simulink model "ignitionScheduler"  (R2024b)
settings: Solver=VariableStepAuto  StartTime=0.0  StopTime=30  RelTol=1e-3
undefined symbols (not defined in the file or in its folder): DOWN_TABLE, DOWN_TH_BP, entity, I, initialize, p0, pressThresh, T, terminate, trigCyl, UP_TABLE, UP_TH_BP
libraries: fl_lib x32, nesl_utility x22, sdl_lib x15, simulink x1, SignalEditorBlockLib x1, engine_lib x1, autolibshared x1
(part 1 of 2)
settings Model: PauseTimes=75  Creator=Guy  LastModifiedBy=isaacito
settings SolverCC: AlgebraicLoopSolver=TrustRegion
settings DataIOCC: ReturnWorkspaceOutputs=off
settings DebuggingCC: UnconnectedInputMsg=warning  UnconnectedOutputMsg=warning  UnconnectedLineMsg=warning  PregeneratedLibrarySubsystemCodeDiagnostic=none  ArithmeticOperatorsInVariantConditions=warning
settings SFSimCC: SimUseLocalCustomCode=off  CustomCodeUndefinedFunction=UseInterfaceOnly
settings RTWCC: RTWUseLocalCustomCode=off  GPUComputeCapability=3.5
settings SimscapeCC: SimscapeNormalizeSystem=off  SimscapeLogType=all  SimscapeLogSimulationStatistics=on  SimscapeLogLimitData=off

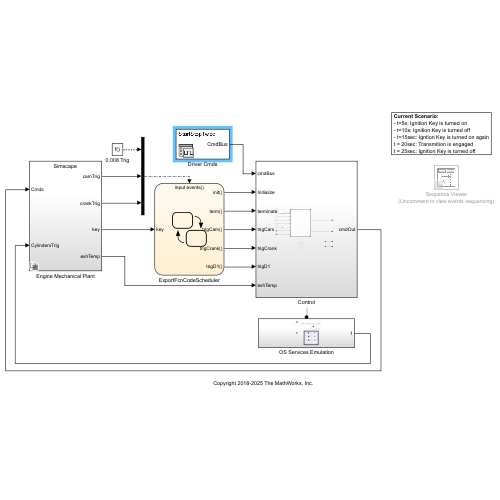
[thumbnail: Simulink's stored preview of the top-level diagram]
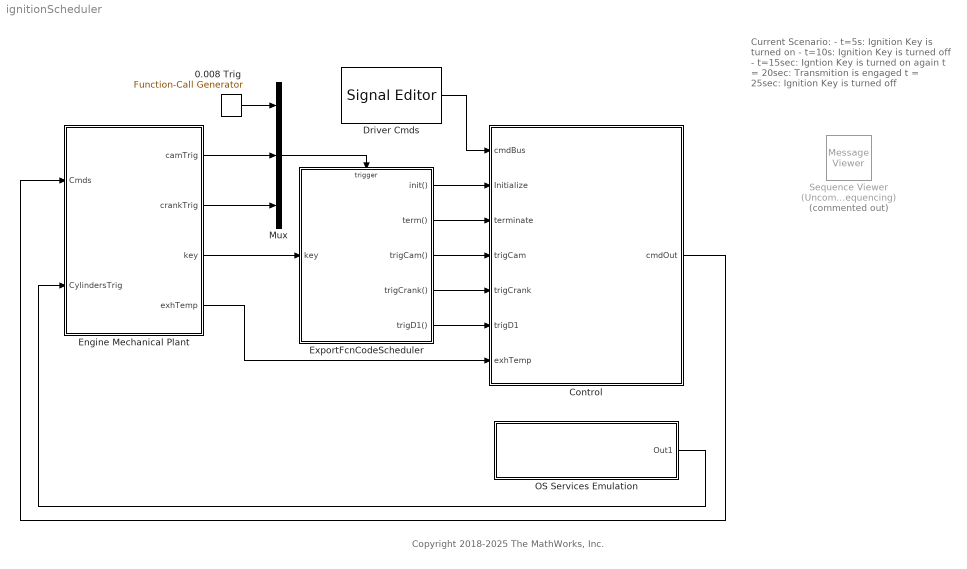
== system ignitionScheduler ==
  note: Current Scenario:
      | - t=5s: Ignition Key is turned on
      | - t=10s: Ignition Key is turned off
      | - t=15sec: Igntion Key is turned on again
      | t = 20sec: Transmition is engaged
      | t = 25sec: Ignition Key is turned off
  note: Copyright 2018-2025 The MathWorks, Inc.
  0.008 Trig : simulink/Ports & Subsystems/Function-Call Generator  sample_time=.008  numberOfIterations=1  DisallowWideOutput=off
  Control : Subsystem  VariantControl=exportFcnCode
  Driver Cmds : SignalEditorBlockLib/Signal Editor  FileName=inputScenarios.mat  ActiveScenario=StartStopTwice  ActiveSignal=CmdBus  IsBus=on  OutputBusObjectStr=Bus: opCmdBus  SampleTime=0  Interpolate=off  ZeroCross=off  OutputAfterFinalValue=Setting to zero  Unit=inherit  PreserveSignalName=on  ApplySigPropsToAllScenarios=on  ApplySigPropsToAllSignals=off
  Engine Mechanical Plant : Subsystem  Variant=on  VariantControlMode=label  LabelModeActiveChoice=SimscapeEngine
  ExportFcnCodeScheduler : Stateflow chart  TreatAsAtomicUnit=on
  Mux : Mux  Inputs=3
  OS Services Emulation : Subsystem
  Sequence Viewer (Uncomment to view events sequencing) : MessageViewer  Commented=on
  wires:
  0.008 Trig/1 -> Mux/1
  Mux/1 -> ExportFcnCodeScheduler/Trigger
  Engine Mechanical Plant/1(camTrig) -> Mux/2
  Engine Mechanical Plant/2(crankTrig) -> Mux/3
  Engine Mechanical Plant/3(key) -> ExportFcnCodeScheduler/1(key)
  Control/1(cmdOut) -> Engine Mechanical Plant/1(Cmds)
  ExportFcnCodeScheduler/1(init()) -> Control/2(Initialize)
  ExportFcnCodeScheduler/2(term()) -> Control/3(terminate)
  ExportFcnCodeScheduler/3(trigCam()) -> Control/4(trigCam)
  ExportFcnCodeScheduler/4(trigCrank()) -> Control/5(trigCrank)
  ExportFcnCodeScheduler/5(trigD1()) -> Control/6(trigD1)
  Engine Mechanical Plant/4(exhTemp) -> Control/7(exhTemp)
  OS Services Emulation/1(Out1) -> Engine Mechanical Plant/2(CylindersTrig)
  Driver Cmds/1 -> Control/1(cmdBus)

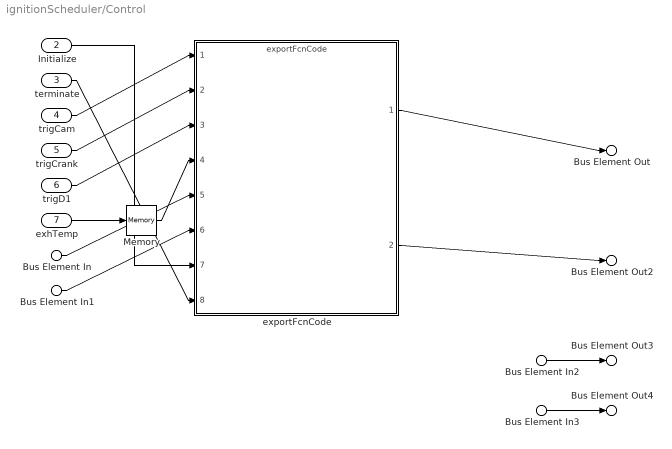
== system ignitionScheduler/Control ==
  Bus Element In1 : Inport  PortName=cmdBus  Element=Throttle
  Bus Element In3 : Inport  PortName=cmdBus  Element=EngageTransmission
  Bus Element In : Inport  PortName=cmdBus  Element=IgnitionKey
  Bus Element In2 : Inport  PortName=cmdBus  Element=IgnitionKey
  Initialize : Inport  Port=2
  terminate : Inport  Port=3
  trigCam : Inport  Port=4
  trigCrank : Inport  Port=5
  trigD1 : Inport  Port=6
  exhTemp : Inport  Port=7
  Memory : Memory
  exportFcnCode : ModelReference  ModelNameDialog=exportFcnCode.slx  SimulationMode=Normal  ShowModelInitializePort=on  ShowModelTerminatePort=on  ScheduleRates=on  ModelEventPortInfo=I:initialize,T:terminate  ModelReferenceVersion=1.150
  Bus Element Out : Outport  VectorParamsAs1DForOutWhenUnconnected=off  PortName=cmdOut  Element=starter
  Bus Element Out2 : Outport  VectorParamsAs1DForOutWhenUnconnected=off  PortName=cmdOut  Element=throttle
  Bus Element Out3 : Outport  VectorParamsAs1DForOutWhenUnconnected=off  PortName=cmdOut  Element=key
  Bus Element Out4 : Outport  VectorParamsAs1DForOutWhenUnconnected=off  PortName=cmdOut  Element=EngageTransmission
  wires:
  exportFcnCode/2 -> Bus Element Out2/1
  exportFcnCode/1 -> Bus Element Out/1
  exhTemp/1 -> Memory/1
  Bus Element In/1 -> exportFcnCode/5
  Bus Element In1/1 -> exportFcnCode/6
  Bus Element In2/1 -> Bus Element Out3/1
  Bus Element In3/1 -> Bus Element Out4/1
  Memory/1 -> exportFcnCode/4
  Initialize/1 -> exportFcnCode/7
  terminate/1 -> exportFcnCode/8
  trigCam/1 -> exportFcnCode/1
  trigCrank/1 -> exportFcnCode/2
  trigD1/1 -> exportFcnCode/3

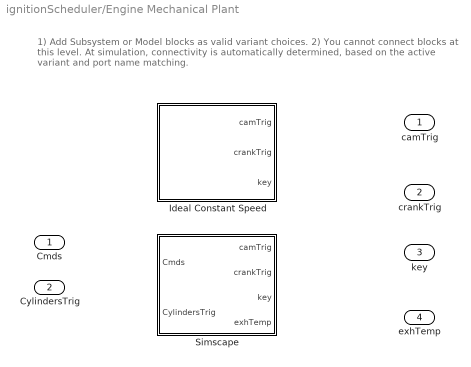
== system ignitionScheduler/Engine Mechanical Plant ==
  note: 1) Add Subsystem or Model blocks as valid variant choices.
      | 2) You cannot connect blocks at this level. At simulation, connectivity is automatically
      | determined, based on the active variant and port name matching.
  Cmds : Inport
  CylindersTrig : Inport  Port=2
  Ideal Constant Speed : Subsystem  VariantControl=idealEngine
  Simscape : Subsystem  VariantControl=SimscapeEngine
  camTrig : Outport  VectorParamsAs1DForOutWhenUnconnected=off
  crankTrig : Outport  Port=2  VectorParamsAs1DForOutWhenUnconnected=off
  key : Outport  Port=3  VectorParamsAs1DForOutWhenUnconnected=off
  exhTemp : Outport  Port=4  VectorParamsAs1DForOutWhenUnconnected=off

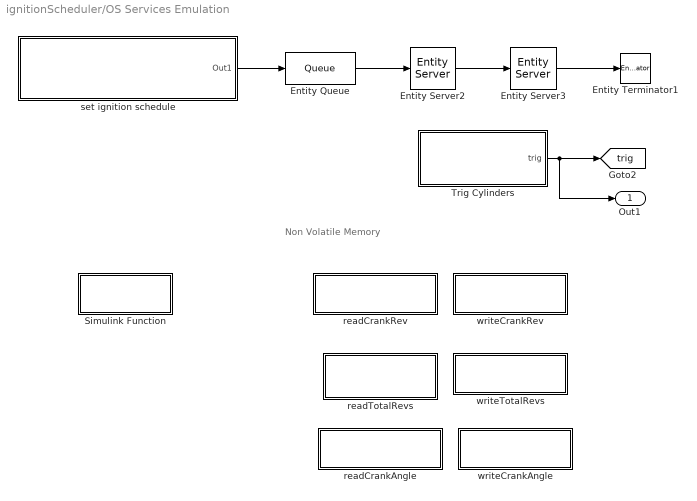
== system ignitionScheduler/OS Services Emulation ==
  note: Non Volatile Memory
  Entity Queue : Queue  InputPortMessageModes=m  OutputPortMessageModes=m  Capacity=1
  Entity Server2 : EntityServer  InputPortMessageModes=m  OutputPortMessageModes=m  Capacity=1  ServiceTimeSource=Attribute  ServiceTimeAttributeName=timeout  ServiceCompleteAction=trigCyl(entity.cyl,true);
  Entity Server3 : EntityServer  InputPortMessageModes=m  OutputPortMessageModes=m  Capacity=1  ServiceTimeSource=Attribute  ServiceTimeValue=0.01  ServiceTimeAttributeName=duration  ServiceCompleteAction=trigCyl(entity.cyl,false);
  Entity Terminator1 : EntityTerminator  InputPortMessageModes=m
  Simulink Function : Subsystem  TreatAsAtomicUnit=on
  Trig Cylinders : Subsystem  TreatAsAtomicUnit=on
  readCrankAngle : Subsystem  TreatAsAtomicUnit=on
  readCrankRev : Subsystem  TreatAsAtomicUnit=on
  readTotalRevs : Subsystem  TreatAsAtomicUnit=on
  set ignition schedule : Subsystem  TreatAsAtomicUnit=on
  writeCrankAngle : Subsystem  TreatAsAtomicUnit=on
  writeCrankRev : Subsystem  TreatAsAtomicUnit=on
  writeTotalRevs : Subsystem  TreatAsAtomicUnit=on
  Out1 : Outport  VectorParamsAs1DForOutWhenUnconnected=off
  tag scope: trig=global
  wires:
  Trig Cylinders/1(trig) -> Out1/1, [trig]
  Entity Server2/1 -> Entity Server3/1
  set ignition schedule/1(Out1) -> Entity Queue/1
  Entity Queue/1 -> Entity Server2/1
  Entity Server3/1 -> Entity Terminator1/1

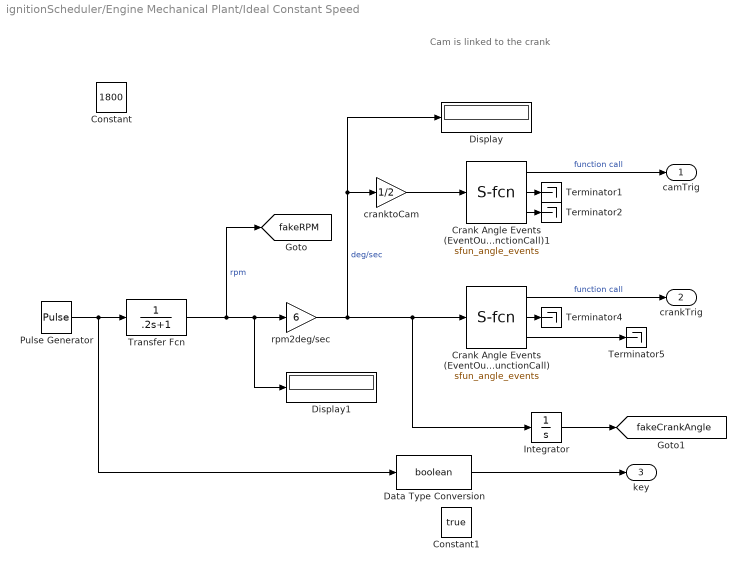
== system ignitionScheduler/Engine Mechanical Plant/Ideal Constant Speed ==
  note: Cam is linked to the crank
  Constant : Constant  Value=1800
  Constant1 : Constant  Value=true  OutDataTypeStr=boolean
  Crank Angle Events (EventOutputType: FunctionCall) : S-Function  LoadFcn=|  FunctionName=sfun_angle_events  Parameters=CrossingAngles, InitialAngle, eventOutputType, clockwiseOnly  SFunctionDeploymentMode=off  EnableBusSupport=off  mask(AnglularIntegratorWithEventDetection){CrossingAngles=[0:10:340], InitialAngle=0, EventOutputType=Function Call, ClockwiseOnly=on}
      | DVG.Registry.registerIcon(...
      | 'BlockIcon.SFunAngleEvents', ...
      | fullfile(matlabroot,'toolbox','simulink','simdemos','simfeatures','slexToothedWheel.svg'))
      mask prompts: CrossingAngles "Crossing Angles:"; InitialAngle "Initial Angle:"; EventOutputType "Event output type:"; ClockwiseOnly "Assume clockwise rotation only"
      mask help:
      | This block integrates the angular velocity input to compute the angle and to fire events at the specified crossing angles. All angles are in degrees, with 0 at the top, incresing clockwise.
      |
      | The crossings angles should be specified as a monotonically increasing vector, with the first element set to 0 and the last element being less than 360 degrees.
      |
      | The first output is a function call, which is fired when an angle crossing event is detected.
      |
      | The second output indicates the direction of the angle crossing event, true for clockwise and false for anti-clockwise.
      |
      | The third output is the angle, wrapped to be in [0, 360) degrees.
      mask init:
      | clockwiseOnly = isequal(get_param(gcb,'ClockwiseOnly'),'on');
      | 
      | switch get_param(gcb,'EventOutputType')
      |     case 'Trigger Pulse'
      |         eventOutputType = 0;
      |     case 'Function Call'
      |         eventOutputType = 1;
      |     otherwise
      |         eventOutputType = 2;
      | end
      mask TypeOptions EventOutputType: Trigger Pulse | Function Call
      mask Display: %image('slexToothedWheel.svg');
  Crank Angle Events (EventOutputType: FunctionCall)1 : S-Function  LoadFcn=|  FunctionName=sfun_angle_events  Parameters=CrossingAngles, InitialAngle, eventOutputType, clockwiseOnly  SFunctionDeploymentMode=off  EnableBusSupport=off  mask(AnglularIntegratorWithEventDetection){CrossingAngles=[0 ], InitialAngle=320, EventOutputType=Function Call, ClockwiseOnly=on}
      | DVG.Registry.registerIcon(...
      | 'BlockIcon.SFunAngleEvents', ...
      | fullfile(matlabroot,'toolbox','simulink','simdemos','simfeatures','slexToothedWheel.svg'))
      mask prompts: CrossingAngles "Crossing Angles:"; InitialAngle "Initial Angle:"; EventOutputType "Event output type:"; ClockwiseOnly "Assume clockwise rotation only"
      mask help:
      | This block integrates the angular velocity input to compute the angle and to fire events at the specified crossing angles. All angles are in degrees, with 0 at the top, incresing clockwise.
      |
      | The crossings angles should be specified as a monotonically increasing vector, with the first element set to 0 and the last element being less than 360 degrees.
      |
      | The first output is a function call, which is fired when an angle crossing event is detected.
      |
      | The second output indicates the direction of the angle crossing event, true for clockwise and false for anti-clockwise.
      |
      | The third output is the angle, wrapped to be in [0, 360) degrees.
      mask init: same as ignitionScheduler/Engine Mechanical Plant/Ideal Constant Speed/Crank Angle Events (EventOutputType: FunctionCall)
      mask TypeOptions EventOutputType: Trigger Pulse | Function Call
      mask Display: %image('slexToothedWheel.svg');
  Data Type Conversion : DataTypeConversion  OutDataTypeStr=boolean  SaturateOnIntegerOverflow=off  RndMeth=Floor
  Display : Display
  Display1 : Display
  Integrator : Integrator  WrapState=on  WrappedStateUpperValue=720  WrappedStateLowerValue=0
  Pulse Generator : DiscretePulseGenerator  PulseType=Time based  Amplitude=1000  Period=100 %6.123  PulseWidth=50  PhaseDelay=1
  Terminator{1..2,4..5} (4 alike) : Terminator
  Transfer Fcn : TransferFcn  Denominator=[.2 1]
  cranktoCam : Gain  Gain=1/2
  rpm2deg/sec : Gain  Gain=6
  camTrig : Outport  VectorParamsAs1DForOutWhenUnconnected=off
  crankTrig : Outport  Port=2  VectorParamsAs1DForOutWhenUnconnected=off
  key : Outport  Port=3  VectorParamsAs1DForOutWhenUnconnected=off
  tag scope: fakeCrankAngle=global, fakeRPM=global
  wires:
  Crank Angle Events (EventOutputType: FunctionCall)1/3 -> Terminator2/1
  Crank Angle Events (EventOutputType: FunctionCall)/3 -> Terminator5/1
  Transfer Fcn/1 -> [fakeRPM], Display1/1, rpm2deg/sec/1  "rpm"
  rpm2deg/sec/1 -> Integrator/1, Crank Angle Events (EventOutputType: FunctionCall)/1, cranktoCam/1, Display/1  "deg/sec"
  Crank Angle Events (EventOutputType: FunctionCall)/2 -> Terminator4/1
  Crank Angle Events (EventOutputType: FunctionCall)/1 -> crankTrig/1  "function call"
  Crank Angle Events (EventOutputType: FunctionCall)1/2 -> Terminator1/1
  cranktoCam/1 -> Crank Angle Events (EventOutputType: FunctionCall)1/1
  Crank Angle Events (EventOutputType: FunctionCall)1/1 -> camTrig/1  "function call"
  Data Type Conversion/1 -> key/1
  Pulse Generator/1 -> Data Type Conversion/1, Transfer Fcn/1
  Integrator/1 -> [fakeCrankAngle]

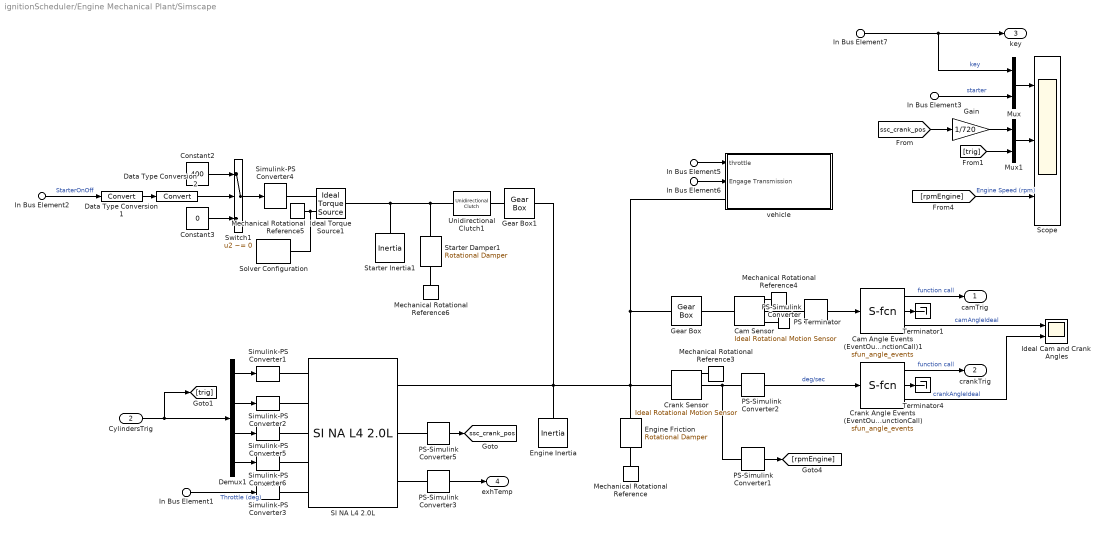
== system ignitionScheduler/Engine Mechanical Plant/Simscape ==
  In Bus Element1 : Inport  PortName=Cmds  Element=throttle
  In Bus Element5 : Inport  PortName=Cmds  Element=throttle
  In Bus Element6 : Inport  PortName=Cmds  Element=EngageTransmission
  In Bus Element7 : Inport  PortName=Cmds  Element=key
  In Bus Element2 : Inport  PortName=Cmds  Element=starter
  In Bus Element3 : Inport  PortName=Cmds  Element=starter
  CylindersTrig : Inport  Port=2
  Cam Angle Events (EventOutputType: FunctionCall)1 : S-Function  LoadFcn=|  FunctionName=sfun_angle_events  Parameters=CrossingAngles, InitialAngle, eventOutputType, clockwiseOnly  SFunctionDeploymentMode=off  EnableBusSupport=off  mask(AnglularIntegratorWithEventDetection){CrossingAngles=[0 ], InitialAngle=320, EventOutputType=Function Call, ClockwiseOnly=on}
      | DVG.Registry.registerIcon(...
      | 'BlockIcon.SFunAngleEvents', ...
      | fullfile(matlabroot,'toolbox','simulink','simdemos','simfeatures','slexToothedWheel.svg'))
      mask prompts: CrossingAngles "Crossing Angles:"; InitialAngle "Initial Angle:"; EventOutputType "Event output type:"; ClockwiseOnly "Assume clockwise rotation only"
      mask help:
      | This block integrates the angular velocity input to compute the angle and to fire events at the specified crossing angles. All angles are in degrees, with 0 at the top, incresing clockwise.
      |
      | The crossings angles should be specified as a monotonically increasing vector, with the first element set to 0 and the last element being less than 360 degrees.
      |
      | The first output is a function call, which is fired when an angle crossing event is detected.
      |
      | The second output indicates the direction of the angle crossing event, true for clockwise and false for anti-clockwise.
      |
      | The third output is the angle, wrapped to be in [0, 360) degrees.
      mask init: same as ignitionScheduler/Engine Mechanical Plant/Ideal Constant Speed/Crank Angle Events (EventOutputType: FunctionCall)
      mask TypeOptions EventOutputType: Trigger Pulse | Function Call
      mask Display: %image('slexToothedWheel.svg');
  Cam Sensor : fl_lib/Mechanical/Mechanical Sensors/Ideal Rotational Motion Sensor  reference=foundation.enum.MeasurementReference.difference  acceleration_port=false  velocity_port=true  position_port=true  wrap_angle=simscape.enum.onoff.off  offset=0 rad
  Constant2 : Constant  Value=400
  Constant3 : Constant  Value=0
  Crank Angle Events (EventOutputType: FunctionCall) : S-Function  LoadFcn=|  FunctionName=sfun_angle_events  Parameters=CrossingAngles, InitialAngle, eventOutputType, clockwiseOnly  SFunctionDeploymentMode=off  EnableBusSupport=off  mask(AnglularIntegratorWithEventDetection){CrossingAngles=[0:10:340], InitialAngle=0, EventOutputType=Function Call, ClockwiseOnly=on}
      | DVG.Registry.registerIcon(...
      | 'BlockIcon.SFunAngleEvents', ...
      | fullfile(matlabroot,'toolbox','simulink','simdemos','simfeatures','slexToothedWheel.svg'))
      mask prompts: CrossingAngles "Crossing Angles:"; InitialAngle "Initial Angle:"; EventOutputType "Event output type:"; ClockwiseOnly "Assume clockwise rotation only"
      mask help:
      | This block integrates the angular velocity input to compute the angle and to fire events at the specified crossing angles. All angles are in degrees, with 0 at the top, incresing clockwise.
      |
      | The crossings angles should be specified as a monotonically increasing vector, with the first element set to 0 and the last element being less than 360 degrees.
      |
      | The first output is a function call, which is fired when an angle crossing event is detected.
      |
      | The second output indicates the direction of the angle crossing event, true for clockwise and false for anti-clockwise.
      |
      | The third output is the angle, wrapped to be in [0, 360) degrees.
      mask init: same as ignitionScheduler/Engine Mechanical Plant/Ideal Constant Speed/Crank Angle Events (EventOutputType: FunctionCall)
      mask TypeOptions EventOutputType: Trigger Pulse | Function Call
      mask Display: %image('slexToothedWheel.svg');
  Crank Sensor : fl_lib/Mechanical/Mechanical Sensors/Ideal Rotational Motion Sensor  reference=foundation.enum.MeasurementReference.difference  acceleration_port=false  velocity_port=true  position_port=true  wrap_angle=simscape.enum.onoff.off  offset=0 rad
  Data Type Conversion1 : DataTypeConversion  SaturateOnIntegerOverflow=off  RndMeth=Floor
  Data Type Conversion2 : DataTypeConversion  SaturateOnIntegerOverflow=off  RndMeth=Floor
  Demux1 : Demux
  Engine Friction : fl_lib/Mechanical/Rotational Elements/Rotational Damper  D=0.06 m*N/rpm  w_specify=off  w_priority=None  w=0 rad/s  w_nominal_specify=off  w_nominal_value=1  w_nominal_unit=rad/s  t_specify=off  t_priority=None  t=0 N*m  t_nominal_specify=off  t_nominal_value=1  t_nominal_unit=N*m
      settings: AttributesFormatString=|
      | %<D>
      | %<D_unit>
  Engine Inertia : fl_lib/Mechanical/Rotational Elements/Inertia  inertia=0.24 kg*m^2  num_ports=foundation.enum.numPorts2.one  w_specify=off  w_priority=High  w=0 rad/s  w_nominal_specify=off  w_nominal_value=1  w_nominal_unit=rad/s  t_specify=off  t_priority=None  t=0 N*m  t_nominal_specify=off  t_nominal_value=1  t_nominal_unit=N*m
      settings: AttributesFormatString=|
      | %<inertia>
      | %<inertia_unit>
      | %<w_specify>
  Gain : Gain  Gain=1/720
  Gear Box : fl_lib/Mechanical/Mechanisms/Gear Box  ratio=2  t_in_specify=off  t_in_priority=None  t_in=0 N*m  t_in_nominal_specify=off  t_in_nominal_value=1  t_in_nominal_unit=N*m  t_out_specify=off  t_out_priority=None  t_out=0 N*m  t_out_nominal_specify=off  t_out_nominal_value=1  t_out_nominal_unit=N*m
  Gear Box1 : fl_lib/Mechanical/Mechanisms/Gear Box  ratio=20  t_in_specify=off  t_in_priority=None  t_in=0 N*m  t_in_nominal_specify=off  t_in_nominal_value=1  t_in_nominal_unit=N*m  t_out_specify=off  t_out_priority=None  t_out=0 N*m  t_out_nominal_specify=off  t_out_nominal_value=1  t_out_nominal_unit=N*m
      settings: AttributesFormatString=%<ratio>
  Ideal Cam and Crank Angles : Scope  NumInputPorts=2
  Ideal Torque Source1 : fl_lib/Mechanical/Mechanical Sources/Ideal Torque Source
  Mechanical Rotational Reference{,3..6} (5 alike) : fl_lib/Mechanical/Rotational Elements/Mechanical Rotational Reference
  Mux : Mux  Inputs=2
  Mux1 : Mux  Inputs=2
  PS Terminator : fl_lib/Physical Signals/Sinks/PS Terminator
  PS-Simulink Converter : nesl_utility/PS-Simulink Converter  PhysicalDomain=network_engine_domain  SubClassName=ps_output  LeftPortType=input  RightPortType=output  PseudoPeriodic=off  Frequencies=[]  VectorFormat=1-D array  Unit=deg/s  AffineConversion=off
  PS-Simulink Converter1 : nesl_utility/PS-Simulink Converter  PhysicalDomain=network_engine_domain  SubClassName=ps_output  LeftPortType=input  RightPortType=output  PseudoPeriodic=off  Frequencies=[]  VectorFormat=1-D array  Unit=rpm  AffineConversion=off
  PS-Simulink Converter2 : nesl_utility/PS-Simulink Converter  PhysicalDomain=network_engine_domain  SubClassName=ps_output  LeftPortType=input  RightPortType=output  PseudoPeriodic=off  Frequencies=[]  VectorFormat=1-D array  Unit=deg/s  AffineConversion=off
  PS-Simulink Converter3 : nesl_utility/PS-Simulink Converter  PhysicalDomain=network_engine_domain  SubClassName=ps_output  LeftPortType=input  RightPortType=output  PseudoPeriodic=off  Frequencies=[]  VectorFormat=1-D array  Unit=degC  AffineConversion=on
  PS-Simulink Converter5 : nesl_utility/PS-Simulink Converter  PhysicalDomain=network_engine_domain  SubClassName=ps_output  LeftPortType=input  RightPortType=output  PseudoPeriodic=off  Frequencies=[]  VectorFormat=1-D array  Unit=deg  AffineConversion=off
  SI NA L4 2.0L : engine_lib/SI NA L4 2.0L
      settings: InternalSimscapePortConfiguration="{\"Bottom\":[],\"Left\":[{\"id\":\"ig1\",\"label\":\"ig1\",\"type\":\"input\"},{\"id\":\"ig2\",\"label\":\"ig2\",\"type\":\"input\"},{\"id\":\"ig3\",\"label\":\"ig3\",\"type\":\"input\"},{\"id\":\"ig4\",\"label\":\"ig4\",\"type\":\"input\"},{\"id\":\"thr_cmd\",\"label\":\"THR\",\"type\":\"input\"}],\"Right\":[{\"id\":\"R\",\"label\":\"R\",\"type\":\"foundation.mechanical.rotational.rotational\"},{\"id\":\"crkpos\",\"label\":\"cpos\",\"type\":\"output\"},{\"id\":\"T_exwall\",\"label\":\"Tew\",\"type\":\"output\"}],\"Top\":[]}"
  Scope : Scope  NumInputPorts=3
  Simulink-PS Converter{1..2,5..6} (4 alike) : nesl_utility/Simulink-PS Converter  PhysicalDomain=network_engine_domain  SubClassName=ps_input  LeftPortType=input  RightPortType=output  PseudoPeriodic=off  Frequencies=[]  NoiseDistribution=none  NoiseParameters=[]  Unit=1  AffineConversion=off  FilteringAndDerivatives=provide  SimscapeFilterOrder=1  InputFilterTimeConstant=0.001  UdotUserProvided=0
  Simulink-PS Converter3 : nesl_utility/Simulink-PS Converter  PhysicalDomain=network_engine_domain  SubClassName=ps_input  LeftPortType=input  RightPortType=output  PseudoPeriodic=off  Frequencies=[]  NoiseDistribution=none  NoiseParameters=[]  Unit=deg  AffineConversion=off  FilteringAndDerivatives=provide  SimscapeFilterOrder=1  InputFilterTimeConstant=0.001  UdotUserProvided=0
  Simulink-PS Converter4 : nesl_utility/Simulink-PS Converter  PhysicalDomain=network_engine_domain  SubClassName=ps_input  LeftPortType=input  RightPortType=output  PseudoPeriodic=off  Frequencies=[]  NoiseDistribution=none  NoiseParameters=[]  Unit=N*m  AffineConversion=off  FilteringAndDerivatives=filter  SimscapeFilterOrder=1  InputFilterTimeConstant=0.001  UdotUserProvided=1
  Solver Configuration : nesl_utility/Solver Configuration  PhysicalDomain=network_engine_domain  SubClassName=solver  LeftPortType=input  RightPortType=generic  Tones=[]  Harmonics=[]  SimulateNoise=off  Profile=off  UseLocalSampling=off  EnableSwitchedLinearOptims=on  FrequencyDomain=off  UseCCode=off  RelTol=0.001  AbsTol=1e-06  MinStep=1e-09  ToWorkspace=off  RevertToSquareIcSolve=off  NumHomotopyIterations=100  PhasorMode=off  PhasorModeNumHarmonics=1  ConsistencySolver=NEWTON_FTOL  IndexReductionMethod=DerivativeReplacement  DoDC=off  ResidualTolerance=1e-09  ConsistencyTolSource=GLOBAL  ConsistencyAbsTol=0.001  ConsistencyRelTol=0.001  ConsistencyTolFactor=0.001  UseLocalSolver=off  LocalSolverChoice=NE_BACKWARD_EULER_ADVANCER  ResolveIndetEquations=on  FunctionEvalNumThread=1  LocalSolverSampleTime=0.001  DoFixedCost=off  MaxNonlinIter=3  MaxModeIter=2  ComputeImpulses=off  ImpulseIterations=2  LinearAlgebra=Sparse  LinearAlgebraNumThread=0  EquationFormulation=NE_TIME_EF  DelaysMemoryBudget=1024  AutomaticFiltering=on  FilteringTimeConstant=0.001  PartitionStorageMethod=AS_NEEDED  PartitionMemoryBudget=1024  PartitionMethod=FAST  MultibodyUseLocalSolver=off  MultibodyLocalSolverChoice=ODE1  MultibodyLocalSolverSampleTime=0.001
      settings: AttributesFormatString=Local solver %<UseLocalSolver>
  Starter Damper1 : fl_lib/Mechanical/Rotational Elements/Rotational Damper  D=0.1 m*N/rpm  w_specify=off  w_priority=None  w=0 rad/s  w_nominal_specify=off  w_nominal_value=1  w_nominal_unit=rad/s  t_specify=off  t_priority=None  t=0 N*m  t_nominal_specify=off  t_nominal_value=1  t_nominal_unit=N*m
      settings: AttributesFormatString=|
      | %<D>
      | %<D_unit>
  Starter Inertia1 : fl_lib/Mechanical/Rotational Elements/Inertia  inertia=30 m^2*g  num_ports=foundation.enum.numPorts2.one  w_specify=off  w_priority=High  w=0 rad/s  w_nominal_specify=off  w_nominal_value=1  w_nominal_unit=rad/s  t_specify=off  t_priority=None  t=0 N*m  t_nominal_specify=off  t_nominal_value=1  t_nominal_unit=N*m
      settings: AttributesFormatString=|
      | %<inertia>
      | %<inertia_unit>
  Switch1 : Switch  Criteria=u2 ~= 0  SaturateOnIntegerOverflow=off  InputSameDT=off
  Terminator1 : Terminator
  Terminator4 : Terminator
  Unidirectional Clutch1 : sdl_lib/Clutches/Unidirectional Clutch  transmission_direction=1  initial_state_locked=0
      settings: InternalSimscapePortConfiguration="{\"Bottom\":[],\"Left\":[{\"id\":\"H\",\"label\":\"H\",\"type\":\"foundation.mechanical.rotational.rotational\"}],\"Right\":[{\"id\":\"R\",\"label\":\"R\",\"type\":\"foundation.mechanical.rotational.rotational\"}],\"Top\":[]}"
  vehicle : Subsystem
  camTrig : Outport  VectorParamsAs1DForOutWhenUnconnected=off
  crankTrig : Outport  Port=2  VectorParamsAs1DForOutWhenUnconnected=off
  key : Outport  Port=3  VectorParamsAs1DForOutWhenUnconnected=off
  exhTemp : Outport  Port=4  VectorParamsAs1DForOutWhenUnconnected=off
  tag scope: ssc_crank_pos=global
  wires:
  Cam Angle Events (EventOutputType: FunctionCall)1/3 -> Ideal Cam and Crank Angles/1  "camAngleIdeal"
  Crank Angle Events (EventOutputType: FunctionCall)/1 -> crankTrig/1  "function call"
  Cam Angle Events (EventOutputType: FunctionCall)1/1 -> camTrig/1  "function call"
  Crank Angle Events (EventOutputType: FunctionCall)/3 -> Ideal Cam and Crank Angles/2  "crankAngleIdeal"
  Cam Angle Events (EventOutputType: FunctionCall)1/2 -> Terminator1/1
  Crank Angle Events (EventOutputType: FunctionCall)/2 -> Terminator4/1
  PS-Simulink Converter/1 -> Cam Angle Events (EventOutputType: FunctionCall)1/1
  PS-Simulink Converter1/1 -> [rpmEngine]
  Mux/1 -> Scope/1
  [rpmEngine] -> Scope/3  "Engine Speed (rpm)"
  PS-Simulink Converter2/1 -> Crank Angle Events (EventOutputType: FunctionCall)/1  "deg/sec"
  CylindersTrig/1 -> [trig], Demux1/1
  Gain/1 -> Mux1/1
  [ssc_crank_pos] -> Gain/1
  [trig] -> Mux1/2
  Mux1/1 -> Scope/2
  In Bus Element3/1 -> Mux/2  "starter"
  In Bus Element5/1 -> vehicle/1(throttle)
  In Bus Element6/1 -> vehicle/2(Engage Transmission)
  In Bus Element7/1 -> Mux/1, key/1  "key"
  In Bus Element1/1 -> Simulink-PS Converter3/1  "Throttle (deg)"
  In Bus Element2/1 -> Data Type Conversion1/1  "StarterOnOff"
  PS-Simulink Converter5/1 -> [ssc_crank_pos]
  PS-Simulink Converter3/1 -> exhTemp/1
  Data Type Conversion1/1 -> Data Type Conversion2/1
  Switch1/1 -> Simulink-PS Converter4/1
  Data Type Conversion2/1 -> Switch1/2
  Constant2/1 -> Switch1/1
  Demux1/3 -> Simulink-PS Converter5/1
  Demux1/1 -> Simulink-PS Converter1/1
  Constant3/1 -> Switch1/3
  Demux1/2 -> Simulink-PS Converter2/1
  Demux1/4 -> Simulink-PS Converter6/1
  connections:
  Mechanical Rotational Reference/LConn1 -- Engine Friction/RConn1
  Gear Box/RConn1 -- Cam Sensor/LConn1
  Mechanical Rotational Reference4/LConn1 -- Cam Sensor/RConn1
  PS-Simulink Converter/LConn1 -- Cam Sensor/RConn2
  PS Terminator/LConn1 -- Cam Sensor/RConn3
  PS-Simulink Converter2/LConn1 -- PS-Simulink Converter1/LConn1 -- Crank Sensor/RConn2
  Mechanical Rotational Reference3/LConn1 -- Crank Sensor/RConn1
  Gear Box1/RConn1 -- SI NA L4 2.0L/RConn1 -- Crank Sensor/LConn1 -- Engine Friction/LConn1 -- vehicle/LConn1 -- Gear Box/LConn1 -- Engine Inertia/LConn1
  Unidirectional Clutch1/LConn1 -- Starter Damper1/LConn1 -- Ideal Torque Source1/LConn1 -- Starter Inertia1/LConn1
  SI NA L4 2.0L/LConn5 -- Simulink-PS Converter3/RConn1
  Mechanical Rotational Reference6/LConn1 -- Starter Damper1/RConn1
  Gear Box1/LConn1 -- Unidirectional Clutch1/RConn1
  Mechanical Rotational Reference5/LConn1 -- Solver Configuration/RConn1 -- Ideal Torque Source1/RConn2
  SI NA L4 2.0L/LConn4 -- Simulink-PS Converter6/RConn1
  SI NA L4 2.0L/RConn2 -- PS-Simulink Converter5/LConn1
  SI NA L4 2.0L/LConn2 -- Simulink-PS Converter2/RConn1
  SI NA L4 2.0L/RConn3 -- PS-Simulink Converter3/LConn1
  SI NA L4 2.0L/LConn1 -- Simulink-PS Converter1/RConn1
  SI NA L4 2.0L/LConn3 -- Simulink-PS Converter5/RConn1
  Ideal Torque Source1/RConn1 -- Simulink-PS Converter4/RConn1

== system ignitionScheduler/OS Services Emulation/Simulink Function ==
  getTime : TriggerPort  TriggerType=function-call  IsSimulinkFunction=on  FunctionName=getTime  VariantControl=(inherit)
  Digital Clock : DigitalClock  SampleTime=-1
  y : ArgOut  DisableCoverage=on  ArgumentName=y
  wires:
  Digital Clock/1 -> y/1

== system ignitionScheduler/OS Services Emulation/Trig Cylinders ==
  trigCyl : TriggerPort  TriggerType=function-call  IsSimulinkFunction=on  FunctionName=trigCyl  FunctionVisibility=scoped  VariantControl=(inherit)
  Assignment : Assignment  DiagnosticForDimensions=Warning  IndexOptions=Index vector (port)  Indices=1  OutputSizes=1
  Constant : Constant  Value=[0 0 0 0]
  cyl : ArgIn  ArgumentName=cyl
  enable : ArgIn  Port=2  ArgumentName=enable
  trig : Outport  VectorParamsAs1DForOutWhenUnconnected=off
  wires:
  Constant/1 -> Assignment/1
  Assignment/1 -> trig/1
  enable/1 -> Assignment/2
  cyl/1 -> Assignment/3

== system ignitionScheduler/OS Services Emulation/readCrankAngle ==
  readCrankAngle : TriggerPort  TriggerType=function-call  IsSimulinkFunction=on  FunctionName=readCrankAngle  VariantControl=(inherit)
  Data Store Read : DataStoreRead  DataStoreName=crankAngle  IndexOptions=Index vector (dialog)  Indices=1  OutputSizes=1
  y : ArgOut  DisableCoverage=on  ArgumentName=y
  wires:
  Data Store Read/1 -> y/1

== system ignitionScheduler/OS Services Emulation/readCrankRev ==
  readCrankRev : TriggerPort  TriggerType=function-call  IsSimulinkFunction=on  FunctionName=readCrankRev  VariantControl=(inherit)
  Data Store Read : DataStoreRead  DataStoreName=rev  IndexOptions=Index vector (dialog)  Indices=1  OutputSizes=1
  y : ArgOut  DisableCoverage=on  OutDataTypeStr=boolean  ArgumentName=y
  wires:
  Data Store Read/1 -> y/1

== system ignitionScheduler/OS Services Emulation/readTotalRevs ==
  readTotalRevs : TriggerPort  TriggerType=function-call  IsSimulinkFunction=on  FunctionName=readTotalRevs  VariantControl=(inherit)
  Data Store Read : DataStoreRead  DataStoreName=totalRevs  IndexOptions=Index vector (dialog)  Indices=1  OutputSizes=1
  y : ArgOut  DisableCoverage=on  ArgumentName=y
  wires:
  Data Store Read/1 -> y/1

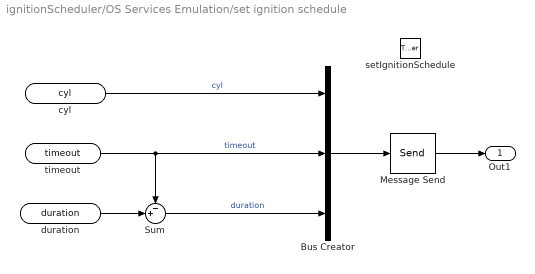
== system ignitionScheduler/OS Services Emulation/set ignition schedule ==
  setIgnitionSchedule : TriggerPort  TriggerType=function-call  IsSimulinkFunction=on  FunctionName=setIgnitionSchedule  VariantControl=(inherit)
  Bus Creator : BusCreator  Inputs=3  OutDataTypeStr=Bus: timerBus  NonVirtualBus=on
  Message Send : Send  OutputPortMessageModes=m
  Sum : Sum  Inputs=-+|
  cyl : ArgIn  ArgumentName=cyl
  timeout : ArgIn  DisableCoverage=on  Port=2  ArgumentName=timeout
  duration : ArgIn  Port=3  ArgumentName=duration
  Out1 : Outport  VectorParamsAs1DForOutWhenUnconnected=off
  wires:
  Message Send/1 -> Out1/1
  cyl/1 -> Bus Creator/1  "cyl"
  Sum/1 -> Bus Creator/3  "duration"
  duration/1 -> Sum/2
  timeout/1 -> Sum/1, Bus Creator/2  "timeout"
  Bus Creator/1 -> Message Send/1

== system ignitionScheduler/OS Services Emulation/writeCrankAngle ==
  writeCrankAngle : TriggerPort  TriggerType=function-call  IsSimulinkFunction=on  FunctionName=writeCrankAngle  VariantControl=(inherit)
  Data Store Write : DataStoreWrite  DataStoreName=crankAngle  IndexOptions=Index vector (dialog)  Indices=1  OutputSizes=1
  u : ArgIn  DisableCoverage=on  ArgumentName=u
  wires:
  u/1 -> Data Store Write/1

== system ignitionScheduler/OS Services Emulation/writeCrankRev ==
  writeCrankRev : TriggerPort  TriggerType=function-call  IsSimulinkFunction=on  FunctionName=writeCrankRev  VariantControl=(inherit)
  Data Store Write : DataStoreWrite  DataStoreName=rev  IndexOptions=Index vector (dialog)  Indices=1  OutputSizes=1
  u : ArgIn  DisableCoverage=on  OutDataTypeStr=boolean  ArgumentName=u
  wires:
  u/1 -> Data Store Write/1

== system ignitionScheduler/OS Services Emulation/writeTotalRevs ==
  writeTotalRevs : TriggerPort  TriggerType=function-call  IsSimulinkFunction=on  FunctionName=writeTotalRevs  VariantControl=(inherit)
  Data Store Write : DataStoreWrite  DataStoreName=totalRevs  IndexOptions=Index vector (dialog)  Indices=1  OutputSizes=1
  u : ArgIn  DisableCoverage=on  ArgumentName=u
  wires:
  u/1 -> Data Store Write/1

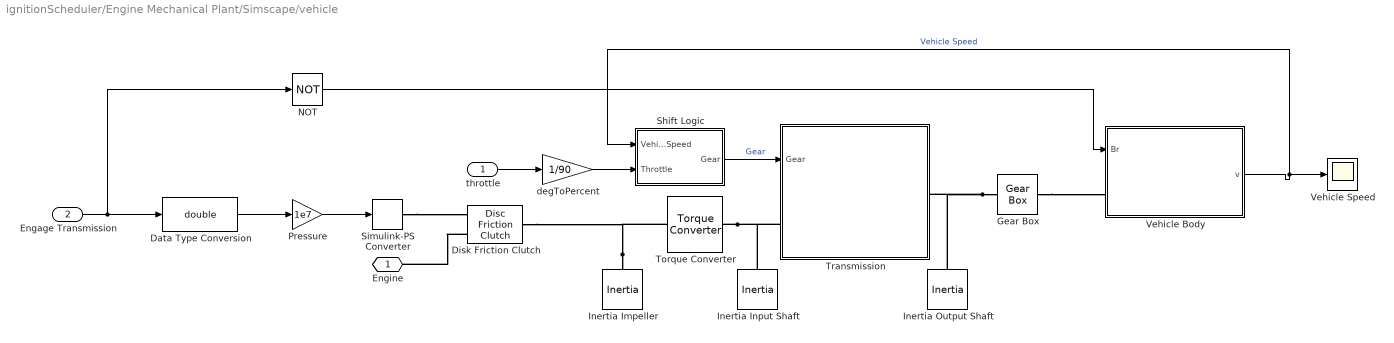
== system ignitionScheduler/Engine Mechanical Plant/Simscape/vehicle ==
  throttle : Inport
  Engage Transmission : Inport  Port=2
  Data Type Conversion : DataTypeConversion  OutDataTypeStr=double  SaturateOnIntegerOverflow=off  RndMeth=Floor
  Disk Friction Clutch : sdl_lib/Clutches/Disc Friction Clutch  geometry_model=1  r_eff=130 mm  d_o=150 mm  d_i=100 mm  nS=4  piston_area=0.001 m^2  unidirectional=0  friction_model=1  mu_w_vector=[0, 100, 1000] rad/s  temperature_TLU=[280, 300, 320] K  mu_static=0.35  mu_static_vector=[.4, .38, .36]  mu_coulomb=0.3  mu_coulomb_vector=[.3, .22, .19]  mu_coulomb_temp_vector=[.3, .28, .25]  mu_coulomb_matrix=[.34, .32, .3; .3, .28, .25; .25, .2, .15]  mu_interp_method=simscape.enum.interpolation.linear  mu_extrap_method=simscape.enum.extrapolation.linear  d_f=1  w_tol=0.001 rad/s  pressure_min=100 Pa  mu_visc=0 N*m/(rad/s)  initial_state_locked=0  thermal_mass=25 kJ/K  T_init=300 K
      settings: InternalSimscapePortConfiguration="{\"Bottom\":[],\"Left\":[{\"id\":\"P\",\"label\":\"P\",\"type\":\"input\"},{\"id\":\"B\",\"label\":\"B\",\"type\":\"foundation.mechanical.rotational.rotational\"}],\"Right\":[{\"id\":\"F\",\"label\":\"F\",\"type\":\"foundation.mechanical.rotational.rotational\"}],\"Top\":[]}"
  Gear Box : fl_lib/Mechanical/Mechanisms/Gear Box  ratio=3  t_in_specify=off  t_in_priority=None  t_in=0 N*m  t_in_nominal_specify=off  t_in_nominal_value=1  t_in_nominal_unit=N*m  t_out_specify=off  t_out_priority=None  t_out=0 N*m  t_out_nominal_specify=off  t_out_nominal_value=1  t_out_nominal_unit=N*m
  Inertia Impeller : fl_lib/Mechanical/Rotational Elements/Inertia  inertia=0.02 kg*m^2  num_ports=foundation.enum.numPorts2.one  w_specify=on  w_priority=High  w=960 rpm  w_nominal_specify=off  w_nominal_value=1  w_nominal_unit=rad/s  t_specify=off  t_priority=High  t=0 N*m  t_nominal_specify=off  t_nominal_value=1  t_nominal_unit=N*m
  Inertia Input Shaft : fl_lib/Mechanical/Rotational Elements/Inertia  inertia=1e-2 kg*m^2  num_ports=foundation.enum.numPorts2.one  w_specify=on  w_priority=High  w=0 rad/s  w_nominal_specify=off  w_nominal_value=1  w_nominal_unit=rad/s  t_specify=off  t_priority=High  t=0 N*m  t_nominal_specify=off  t_nominal_value=1  t_nominal_unit=N*m
  Inertia Output Shaft : fl_lib/Mechanical/Rotational Elements/Inertia  inertia=1e-1 kg*m^2  num_ports=foundation.enum.numPorts2.one  w_specify=on  w_priority=High  w=0 rad/s  w_nominal_specify=off  w_nominal_value=1  w_nominal_unit=rad/s  t_specify=off  t_priority=High  t=0 N*m  t_nominal_specify=off  t_nominal_value=1  t_nominal_unit=N*m
  NOT : Logic  Operator=NOT  IconShape=distinctive  AllPortsSameDT=off  OutDataTypeStr=boolean
  Pressure : Gain  Gain=1e7
  Shift Logic : Stateflow chart  Tag=PublishSubsystem  TreatAsAtomicUnit=on
  Simulink-PS Converter : nesl_utility/Simulink-PS Converter  PhysicalDomain=network_engine_domain  SubClassName=ps_input  LeftPortType=input  RightPortType=output  PseudoPeriodic=off  Frequencies=[]  NoiseDistribution=none  NoiseParameters=[]  Unit=1  AffineConversion=off  FilteringAndDerivatives=filter  SimscapeFilterOrder=2  InputFilterTimeConstant=.5  UdotUserProvided=0
  Torque Converter : sdl_lib/Couplings & Drives/Torque Converter  coast_mode_modeling=sdl.enum.torqueConverterContinuousTwomode.continuous  SR_drive_tlu=[0, .5, .6, .7, .8, .87, .92, .94, .96, .97, 1]  TR_drive_tlu=[2.232, 1.5462, 1.4058, 1.2746, 1.1528, 1.0732, 1.0192, 1, 1, 1, 1]  CF_drive_tlu=1e-4 * [.72558, .66322, .63463, .59042, .51331, .4144, .29287, .22444, .12186, .04386, 0] N*m/rpm^2  SR_coast_tlu=[0, .5, .6, .7, .8, .87, .92, .94, .96, .97, 1]  CF_coast_tlu=1e-4 * [.5079, .4643, .4442, .4133, .3593, .2901, .205, .1571, .0853, .0307, 0] N*m/rpm^2  iniMode=sdl.enum.torqueConverterInitialMode.drive  delta_w=1 rpm  n_vector=[0 0.50 0.60 0.70 0.80 0.87 0.92 0.94 0.96 0.97]  trq_vector="0.999*[10   2.0000    1.6667    1.4286    1.2500    1.1494    1.0870    1.0638    1.0417    1.0309]"  cf_vector_parameterization=1  cf_vector_reference_speed=1  cf_vector=[12.2938 12.8588 13.1452 13.6285 14.6163 16.2675 19.3503 22.1046 29.9986 50.00] (rad/s)/(N*m)^0.5  cf_vector_sq=1e-3*[ 6.616 6.048 5.787 5.384 4.681 3.779 2.671 2.047 1.111 0.400] N*m/(rad/s)^2  interp_method=simscape.enum.interpolation.linear  extrap_method=simscape.enum.extrapolation.linear  model_lag=0  tau=0.02 s  initial_trq_ratio=0
      settings: InternalSimscapePortConfiguration="{\"Bottom\":[],\"Left\":[{\"id\":\"I\",\"label\":\"I\",\"type\":\"foundation.mechanical.rotational.rotational\"}],\"Right\":[{\"id\":\"T\",\"label\":\"T\",\"type\":\"foundation.mechanical.rotational.rotational\"}],\"Top\":[]}"
  Transmission : Subsystem  Tag=PublishSubsystem  mask(CR-CR 4-Speed){}
      mask help: This is a template for a CR-CR 4-speed transmission. Copy it to your model, open it as a subsystem, and modify it for your use.
      settings: OpenFcn=open_system(gcbh,'force');
      mask Display:
      | % Icon data
      | Icon.x1 = [-1.3 -1.1 -1.1 -1 -1 -1 -0.9 -0.9 -0.9 -0.8 -0.8];
      | Icon.x1_1 = [-0.8 -0.7 -0.7 -0.7 -0.6 -0.6 -0.6 -0.5 -0.5 -0.5];
      | Icon.y1 = [0 0 0.15 0.15 0.05 0.15 0.15 0.05 0.15 0.15 0.05];
      | Icon.y1_1 =[0.15 0.15 0.05 0.15 0.15 0.07 0.15 0.15 0.07 0.15];
      | Icon.x2 = [-1.05 -1.05 -0.95 -0.95 -0.95 0.3];
      | Icon.y2 = [0.08   0     0     0.08  0    0];
      | Icon.x3 = [-0.85 -0.85 -0.75 -0.75 -0.75 0 0 -0.3 -0.3  0.3];
      | Icon.y3 = [0.08 0.02 0.02 0.08 0.02 0.02 0.15 0.15 0.33 0.33];
      | Icon.x3_1 = [-0.65 -0.65 -0.55 -0.55 -0.55 -0.4];
      | Icon.y3_1 = [0.1    0.05  0.05  0.1   0.05 0.05];
      | Icon.x4 = [-0.2 -0.1 -0.15 -0.15 -0.2 -0.1];
      | Icon.y4 = [0.12 0.12 0.12 0.18 0.18 0.18];
      | Icon.x5 = [-0.2 -0.1 -0.1 -0.15 -0.15 -0.4 -0.4];
      | Icon.y5 = [0.1 0.1 0.1 0.1 0.05 0.05 0.4];
      | Icon.x6 = [-0.2 -0.1 -0.15 -0.15 0.1 0.1 0.4 0.4];
      | Icon.y6 = [0.20 0.20 0.20 0.3 0.3 0.19 0.19 0];
      | Icon.x7 = [0.3 0.3 0.25 0.35];
      | Icon.y7 = [0 0.13 0.13 0.13];
      | Icon.x8 = [0.25 0.35 0.3 0.3 0.25 0.35];
      | Icon.y8 = [0.15 0.15 0.15 0.23 0.23 0.23];
      | Icon.x9 = [0.25 0.35 0.3 0.3];
      | Icon.y9 = [0.25 0.25 0.25 0.40];
      | Icon.x10 = [0.25 0.25 0.35 0.35 0.35 0.15 0.15 0.15];
      | Icon.y10 = [0.35 0.45 0.45 0.35 0.45 0.45 0.35 0.45];
      | Icon.x11 = [0.2 0.2];
      | Icon.y11 = [0.33 0.40];
      | Icon.x12 = [0.4 0.6];
      | Icon.y12 = [0 0];
      | Icon.x13 = [-0.45 -0.45 -0.35 -0.35 -0.35 -0.55 -0.55];
      | Icon.y13 = [0.35 0.45 0.45 0.35 0.45 0.45 0.35];
      | Icon.x14 = [-0.4 -0.5 -0.5];
      | Icon.y14 = [0.33 0.33 0.4];
      | Icon.x15 = [-0.5 0.35];
      | Icon.y15 = [0.45 0.45];
      | Icon.x16 = [-1.3 -1.1 -1.1 -1 -1 -1 -0.9 -0.9 ];
      | Icon.x16_1 = [-0.9 -0.8 -0.8 -0.8 -0.7 -0.7 -0.7 -0.6];
      | Icon.x16_2 = [-0.6 -0.6 -0.5 -0.5 -0.5];
      | Icon.y16 = [0 0 -0.15 -0.15 -0.05 -0.15 -0.15 -0.05];
      | Icon.y16_1 = [-0.15 -0.15 -0.05 -0.15 -0.15 -0.05 -0.15 -0.15];
      | Icon.y16_2 = [-0.07 -0.15 -0.15 -0.07 -0.15];
      | Icon.x17 = [-1.05 -1.05 -0.95 -0.95 -0.95 0.3];
      | Icon.y17 = [-0.08 0 0 -0.08 0 0];
      | Icon.x18 = [-0.85 -0.85 -0.75 -0.75 -0.75 0 0 -0.3];
      | Icon.x18_1 = [-0.3  0.3];
      | Icon.x18_2 = [-0.65 -0.65 -0.55 -0.55 -0.55 -0.4];
      | Icon.y18 = [-0.08 -0.02 -0.02 -0.08 -0.02 -0.02 -0.15 -0.15];
      | Icon.y18_1 = [-0.33 -0.33];
      | Icon.y18_2 = [-0.1 -0.05 -0.05 -0.1 -0.05 -0.05];
      | Icon.x19 = [-0.2 -0.1 -0.15 -0.15 -0.2 -0.1];
      | Icon.y19 = [-0.12 -0.12 -0.12 -0.18 -0.18 -0.18];
      | Icon.x20 = [-0.2 -0.1 -0.1 -0.15 -0.15 -0.4 -0.4];
      | Icon.y20 = [-0.1 -0.1 -0.1 -0.1 -0.05 -0.05 -0.4];
      | Icon.x21 = [-0.2 -0.1 -0.15 -0.15 0.1 0.1 0.4 0.4];
      | Icon.y21 = [-0.20 -0.20 -0.20 -0.3 -0.3 -0.19 -0.19 0];
      | Icon.x22 = [0.3 0.3 0.25 0.35];
      | Icon.y22 = [0 -0.13 -0.13 -0.13];
      | Icon.x23 = [0.25 0.35 0.3 0.3 0.25 0.35];
      | Icon.y23 = [-0.15 -0.15 -0.15 -0.23 -0.23 -0.23];
      | Icon.x24 = [0.25 0.35 0.3 0.3];
      | Icon.y24 = [-0.25 -0.25 -0.25 -0.40];
      | Icon.x25 = [0.25 0.25 0.35 0.35 0.35 0.15 0.15 0.15];
      | Icon.y25 = [-0.35 -0.45 -0.45 -0.35 -0.45 -0.45 -0.35 -0.45];
      | Icon.x26 = [0.2 0.2];
      | Icon.y26 = [-0.33 -0.40];
      | Icon.x27 = [-0.45 -0.45 -0.35 -0.35 -0.35 -0.55 -0.55];
      | Icon.y27 = [-0.35 -0.45 -0.45 -0.35 -0.45 -0.45 -0.35];
      | Icon.x28 = [-0.4 -0.5 -0.5];
      | Icon.y28 = [-0.33 -0.33 -0.4];
      | Icon.x29 = [-0.5 0.35];
      | Icon.y29 = [-0.45 -0.45];
      | % Bounding box
      | Icon.LowerLeftx = -1.4;
      | Icon.LowerLefty = -0.55;
      | Icon.UpperRightx = 1.0;
      | Icon.UpperRighty = 0.55;
      | 
      | plot(Icon.x1,Icon.y1);
      | plot(Icon.x1_1,Icon.y1_1);
      | plot(Icon.x2,Icon.y2);
      | plot(Icon.x3,Icon.y3);
      | plot(Icon.x3_1,Icon.y3_1);
      | plot(Icon.x4,Icon.y4);
      | plot(Icon.x5,Icon.y5);
      | plot(Icon.x6,Icon.y6);
      | plot(Icon.x7,Icon.y7);
      | plot(Icon.x8,Icon.y8);
      | plot(Icon.x9,Icon.y9);
      | plot(Icon.x10,Icon.y10);
      | plot(Icon.x11,Icon.y11);
      | plot(Icon.x12,Icon.y12);
      | plot(Icon.x13,Icon.y13);
      | plot(Icon.x14,Icon.y14);
      | plot(Icon.x15,Icon.y15);
      | plot(Icon.x16,Icon.y16);
      | plot(Icon.x16_1,Icon.y16_1);
      | plot(Icon.x16_2,Icon.y16_2);
      | plot(Icon.x17,Icon.y17);
      | plot(Icon.x18,Icon.y18);
      | plot(Icon.x18_1,Icon.y18_1);
      | plot(Icon.x18_2,Icon.y18_2);
      | plot(Icon.x19,Icon.y19);
      | plot(Icon.x20,Icon.y20);
      | plot(Icon.x21,Icon.y21);
      | plot(Icon.x22,Icon.y22);
      | plot(Icon.x23,Icon.y23);
      | plot(Icon.x24,Icon.y24);
      | plot(Icon.x25,Icon.y25);
      | plot(Icon.x26,Icon.y26);
      | plot(Icon.x27,Icon.y27);
      | plot(Icon.x28,Icon.y28);
      | plot(Icon.x29,Icon.y29);
      | 
      | plot(Icon.LowerLeftx,Icon.LowerLefty);
      | plot(Icon.UpperRightx,Icon.UpperRighty);
  Vehicle Speed : Scope
  Vehicle Body : Subsystem  Variant=on  VariantControlMode=label  VariantControl=Variant1  LabelModeActiveChoice=Simscape
      mask Display:
      | color('white')
      | plot(-120,-60); plot(120,50);
      | color('black')
      | plot(sin(0:0.1:6*pi)*15-70,cos(0:0.1:6*pi)*15-30);
      | plot(sin(0:0.1:6*pi)*15+70,cos(0:0.1:6*pi)*15-30);
      | plot([-88 -95 -99 -99 -95 -75 -65 -50 -46 10 30 34 80 85 90 93 95 93 90 88],[-30 -28 -23 -5 0 5 10 20 21 21 0 -2 -7 -9 -13 -17 -25 -28 -30 -30])
      | plot([-88 -95 -99 -99 -95 -75 -65 -50 -46 10 30 34 80 85 90 93 95 93 90 88],[-30 -28 -23 -5 0 5 10 20 21 21 0 -2 -7 -9 -13 -17 -25 -28 -30 -30]-1)
      | plot([-88 -95 -99 -99 -95 -75 -65 -50 -46 10 30 34 80 85 90 93 95 93 90 88]+1,[-30 -28 -23 -5 0 5 10 20 21 21 0 -2 -7 -9 -13 -17 -25 -28 -30 -30])
      | plot([-50 50],[-30 -30])
  degToPercent : Gain  Gain=1/90
  Engine : PMIOPort  Side=Left
  wires:
  Pressure/1 -> Simulink-PS Converter/1
  Vehicle Body/1(" v") -> Shift Logic/1(VehicleSpeed), Vehicle Speed/1  "Vehicle Speed"
  Engage Transmission/1 -> NOT/1, Data Type Conversion/1
  Data Type Conversion/1 -> Pressure/1
  Shift Logic/1(Gear) -> Transmission/1(Gear)  "Gear"
  degToPercent/1 -> Shift Logic/2(Throttle)
  NOT/1 -> Vehicle Body/1("Br ")
  throttle/1 -> degToPercent/1
  connections:
  Gear Box/LConn1 -- Inertia Output Shaft/LConn1 -- Transmission/RConn1
  Inertia Impeller/LConn1 -- Disk Friction Clutch/RConn1 -- Torque Converter/LConn1
  Torque Converter/RConn1 -- Transmission/LConn1 -- Inertia Input Shaft/LConn1
  Gear Box/RConn1 -- Vehicle Body/LConn1
  Simulink-PS Converter/RConn1 -- Disk Friction Clutch/LConn1
  Disk Friction Clutch/LConn2 -- Engine/RConn1

== system ignitionScheduler/Engine Mechanical Plant/Simscape/vehicle/Shift Logic/ComputeThreshold ==
  note: Threshold Calculation
  Gear : Inport
  Throttle : Inport  Port=2
  f : TriggerPort  TriggerType=function-call  VariantControl=Variant
      settings: CopyFcn=Stateflow.SLINSF.SimulinkMan.removeBlockPreDeleteFcn  PreDeleteFcn=Stateflow.SLINSF.SimulinkMan.unsafePredeleteFcn
  InterpDown : Lookup_n-D  LookupTableObject=''  BreakpointsForDimension1=DOWN_TH_BP  BreakpointsForDimension2=[1:4]  Table=DOWN_TABLE  OutDataTypeStr=double  InputSameDT=off  LockScale=on
      settings: InputPortMap=u0,u1
  InterpUp : Lookup_n-D  LookupTableObject=''  BreakpointsForDimension1=UP_TH_BP  BreakpointsForDimension2=[1,2,3,4]  Table=UP_TABLE  OutDataTypeStr=double  InputSameDT=off  LockScale=on
      settings: InputPortMap=u0,u1
  down_th : Outport  InitialOutput=0  VectorParamsAs1DForOutWhenUnconnected=off
  up_th : Outport  Port=2  InitialOutput=0  VectorParamsAs1DForOutWhenUnconnected=off
  wires:
  Gear/1 -> InterpUp/2, InterpDown/2
  Throttle/1 -> InterpUp/1, InterpDown/1
  InterpDown/1 -> down_th/1
  InterpUp/1 -> up_th/1
